simulink model "Inverse_Dynamic_Control"  (Simulink 9.2)
settings: Solver=VariableStepAuto  StartTime=0.0  StopTime=4  RelTol=1e-3
undefined symbols (not defined in the file or in its folder): DiscIntNeverNeededParam, q0, q0_dot, Tc
settings Model: Creator=sujay  LastModifiedBy=sujay
settings DataIOCC: LimitDataPoints=off  SaveFormat=Dataset  SignalLoggingSaveFormat=Dataset  ReturnWorkspaceOutputs=on
settings OptimizationCC: LifeSpan=auto
settings DebuggingCC: UnderspecifiedInitializationDetection=Simplified  MergeDetectMultiDrivingBlocksExec=error  FcnCallInpInsideContextMsg=error  StateNameClashWarn=none  SFUnexpectedBacktrackingDiag=error  SFNoUnconditionalDefaultTransitionDiag=error  SFExecutionAtInitializationDiag=warning
settings HardwareCC: ProdBitPerPointer=64  ProdBitPerSizeT=64  ProdBitPerPtrDiffT=64  ProdLargestAtomicFloat=Float  ProdIntDivRoundTo=Zero  ProdEndianess=LittleEndian  ProdWordSize=64  ProdHWDeviceType=Intel->x86-64 (Windows64)
settings ModelReferenceCC: PropagateSignalLabelsOutOfModel=on
settings SFSimCC: SimUseLocalCustomCode=on
settings RTWCC: RTWUseLocalCustomCode=on
settings CodeAppCC: StateflowObjectComments=off
settings GRTTargetCC: TargetLangStandard=C99 (ISO)  GeneratePreprocessorConditionals=Use local settings  CombineOutputUpdateFcns=on  GRTInterface=off
settings ConfigComp: CovMetricSettings=dwe  CovHtmlReporting=off  CovSaveCumulativeToWorkspaceVar=off  CovSaveSingleToWorkspaceVar=off  CovExternalEMLEnable=on

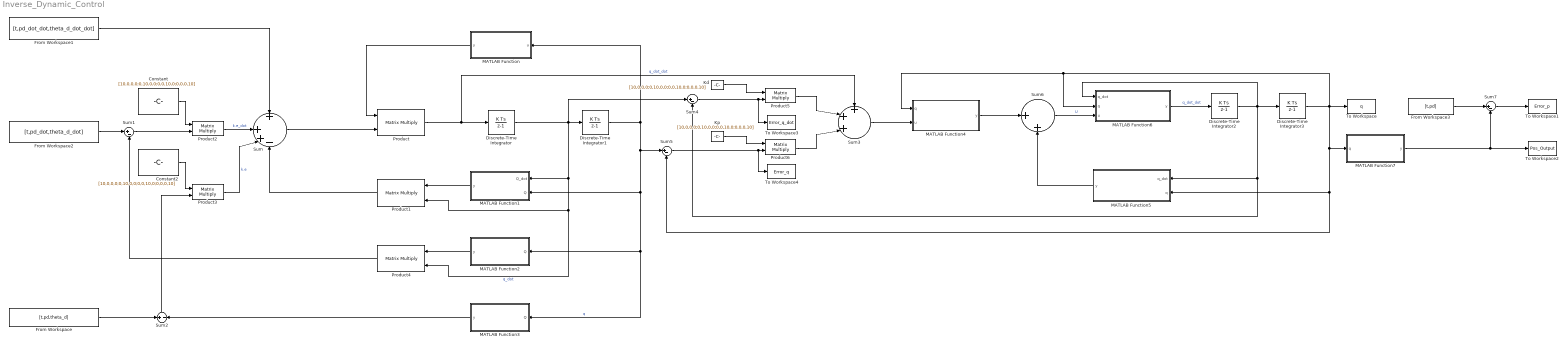
== system Inverse_Dynamic_Control ==
  Constant : Constant  Value=[10,0,0,0;0,10,0,0;0,0,10,0;0,0,0,10]  VectorParams1D=off
  Constant2 : Constant  Value=[10,0,0,0;0,10,0,0;0,0,10,0;0,0,0,10]  VectorParams1D=off
  Discrete-Time Integrator : DiscreteIntegrator  InitialCondition=q0_dot  SampleTime=Tc  ICPrevOutput=DiscIntNeverNeededParam  ICPrevScaledInput=DiscIntNeverNeededParam
  Discrete-Time Integrator1 : DiscreteIntegrator  InitialCondition=q0  SampleTime=Tc  ICPrevOutput=DiscIntNeverNeededParam  ICPrevScaledInput=DiscIntNeverNeededParam
  Discrete-Time Integrator2 : DiscreteIntegrator  InitialCondition=q0_dot  SampleTime=Tc  ICPrevOutput=DiscIntNeverNeededParam  ICPrevScaledInput=DiscIntNeverNeededParam
  Discrete-Time Integrator3 : DiscreteIntegrator  InitialCondition=q0  SampleTime=Tc  ICPrevOutput=DiscIntNeverNeededParam  ICPrevScaledInput=DiscIntNeverNeededParam
  From Workspace : FromWorkspace  VariableName=[t,pd,theta_d]  SampleTime=0
  From Workspace1 : FromWorkspace  VariableName=[t,pd_dot_dot,theta_d_dot_dot]  SampleTime=0
  From Workspace2 : FromWorkspace  VariableName=[t,pd_dot,theta_d_dot]  SampleTime=0
  From Workspace3 : FromWorkspace  VariableName=[t,pd]  SampleTime=0
  Kd : Constant  Value=[10,0,0,0;0,10,0,0;0,0,10,0;0,0,0,10]  VectorParams1D=off
  Kp : Constant  Value=[10,0,0,0;0,10,0,0;0,0,10,0;0,0,0,10]  VectorParams1D=off
  MATLAB Function : MATLAB Function  TreatAsAtomicUnit=on
  MATLAB Function1 : MATLAB Function  TreatAsAtomicUnit=on
  MATLAB Function2 : MATLAB Function  TreatAsAtomicUnit=on
  MATLAB Function3 : MATLAB Function  TreatAsAtomicUnit=on
  MATLAB Function4 : MATLAB Function  TreatAsAtomicUnit=on
  MATLAB Function5 : MATLAB Function  TreatAsAtomicUnit=on
  MATLAB Function6 : MATLAB Function  TreatAsAtomicUnit=on
  MATLAB Function7 : MATLAB Function  TreatAsAtomicUnit=on
  Product{,1..6} (7 alike) : Product  Multiplication=Matrix(*)
  Sum : Sum  Inputs=+|++-
  Sum{1,4..5,7} (4 alike) : Sum  Inputs=|+-
  Sum2 : Sum  Inputs=+|-
  Sum3 : Sum  Inputs=+++|
  Sum6 : Sum  Inputs=|++
  To Workspace : ToWorkspace  VariableName=q  SampleTime=-1
  To Workspace1 : ToWorkspace  VariableName=Error_p  SampleTime=-1
  To Workspace2 : ToWorkspace  VariableName=Pos_Output  SampleTime=-1
  To Workspace3 : ToWorkspace  VariableName=Error_q_dot  SampleTime=-1
  To Workspace4 : ToWorkspace  VariableName=Error_q  SampleTime=-1
  wires:
  From Workspace2/1 -> Sum1/1
  Product4/1 -> Sum1/2
  MATLAB Function1/1(y) -> Product1/1
  Discrete-Time Integrator1/1 -> MATLAB Function2/1(Q), MATLAB Function3/1(Q), MATLAB Function1/2(Q), Sum5/1, MATLAB Function/1(u)  "q"
  Constant/1 -> Product2/1
  MATLAB Function/1(y) -> Product/1
  Sum1/1 -> Product2/2
  Sum2/1 -> Product3/2
  Constant2/1 -> Product3/1
  Product3/1 -> Sum/3  "k.e"
  From Workspace/1 -> Sum2/1
  MATLAB Function2/1(y) -> Product4/1
  MATLAB Function3/1(y) -> Sum2/2
  Product2/1 -> Sum/2  "k.e_dot"
  Sum/1 -> Product/2
  From Workspace1/1 -> Sum/1
  Product1/1 -> Sum/4
  Product/1 -> Discrete-Time Integrator/1, Sum3/1  "q_dot_dot"
  Discrete-Time Integrator/1 -> Sum4/1, Product1/2, Product4/2, MATLAB Function1/1(Q_dot), Discrete-Time Integrator1/1  "q_dot"
  Kd/1 -> Product5/1
  Sum4/1 -> To Workspace3/1, Product5/2
  Product5/1 -> Sum3/2
  Sum5/1 -> To Workspace4/1, Product6/2
  Kp/1 -> Product6/1
  Product6/1 -> Sum3/3
  Sum3/1 -> MATLAB Function4/2(u)
  MATLAB Function4/1(y) -> Sum6/1
  MATLAB Function5/1(y) -> Sum6/2
  Discrete-Time Integrator3/1 -> To Workspace/1, Sum5/2, MATLAB Function5/2(q), MATLAB Function7/1(q), MATLAB Function6/2(q), MATLAB Function4/1(q)
  Sum6/1 -> MATLAB Function6/3(u)  "U"
  MATLAB Function6/1(y) -> Discrete-Time Integrator2/1  "q_dot_dot"
  Discrete-Time Integrator2/1 -> MATLAB Function6/1(q_dot), MATLAB Function5/1(q_dot), Sum4/2, Discrete-Time Integrator3/1
  From Workspace3/1 -> Sum7/1
  MATLAB Function7/1(y) -> To Workspace2/1, Sum7/2
  Sum7/1 -> To Workspace1/1

== matlab function MATLAB Function1 ==
  data: Q_dot input double; Q input double; y output double
function y = Jacobian_dot(Q_dot,Q)
y = Jacobian_dot(Q,Q_dot);
end

== matlab function MATLAB Function ==
  data: u input double; y output double
function y = Inverse_Jacobian(u)
y = inv(Jacobian(u));
end

== matlab function MATLAB Function2 ==
  data: Q input double; y output double
function y = jacobian(Q)
y = Jacobian(Q);
end

== matlab function MATLAB Function3 ==
  data: Q input double; y output double
function y = Kinematics(Q)
y = [ 0.5*(cos(Q(1,1)+Q(2,1))+cos(Q(1,1))) ; 0.5*(sin(Q(1,1)+Q(2,1))+sin(Q(1,1))) ; (1 - Q(3,1)) ; Q(1,1)+Q(2,1)+Q(4,1) ];
end

== matlab function MATLAB Function4 ==
  data: q input double; u input double; y output double
function y = B_q(q,u)

y = B(q)*u;

end

== matlab function MATLAB Function5 ==
  data: q_dot input double; y output double; q input double
function y = n_q_qdot(q_dot,q)

y = n(q,q_dot);

end

== matlab function MATLAB Function6 ==
  data: q_dot input double; q input double; u input double; y output double
function y = Manipulator(q_dot,q,u)

y = dynamic_model(q_dot,q,u);

end

== matlab function MATLAB Function7 ==
  data: q input double; y output double
function y = Kinematics_P(q)
y = [ 0.5*(cos(q(1,1)+q(2,1))+cos(q(1,1))) ; 0.5*(sin(q(1,1)+q(2,1))+sin(q(1,1))) ; (1 - q(3,1)) ];
end
